simulink model "HeltonNonlinearProjectOne"  (R2018a)
settings: Solver=VariableStepAuto  StartTime=0.0  StopTime=100  MinStep=.001  RelTol=1e-5
settings Model: Creator=J  LastModifiedBy=J

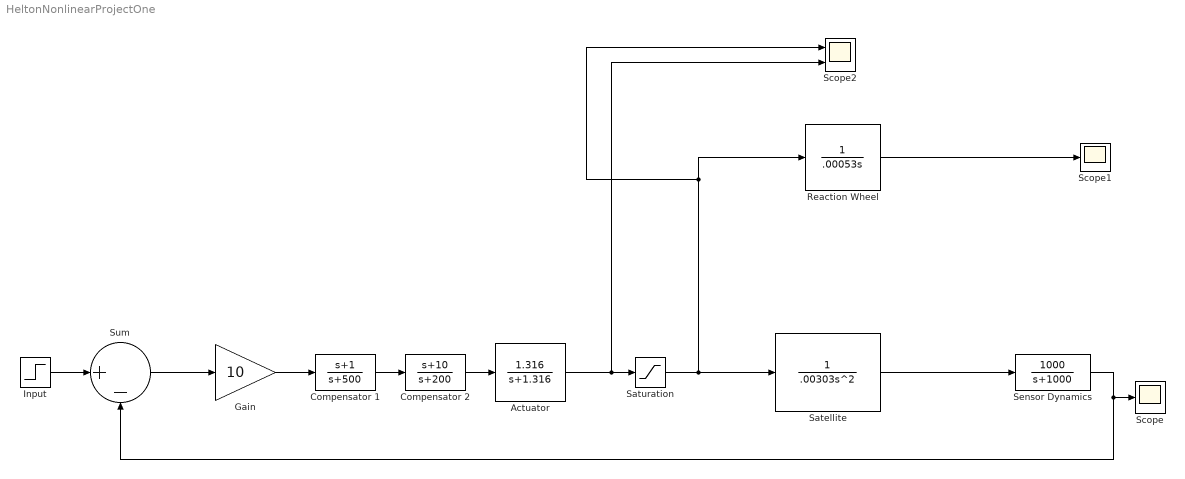
== system HeltonNonlinearProjectOne ==
  Actuator : TransferFcn  Numerator=[1.316]  Denominator=[1 1.316]
  Compensator 1 : TransferFcn  Numerator=[1 1]  Denominator=[1 500]
  Compensator 2 : TransferFcn  Numerator=[1 10]  Denominator=[1 200]
  Gain : Gain  Gain=10
  Input : Step  SampleTime=0
  Reaction Wheel : TransferFcn  Denominator=[.00053 0]
  Satellite : TransferFcn  Denominator=[.00303 0 0]
  Saturation : Saturate  UpperLimit=0.007  LowerLimit=-0.007
  Scope : Scope
  Scope1 : Scope
  Scope2 : Scope  NumInputPorts=2
  Sensor Dynamics : TransferFcn  Numerator=[1000]  Denominator=[1 1000]
  Sum : Sum  Inputs=|+-
  wires:
  Sum/1 -> Gain/1
  Input/1 -> Sum/1
  Reaction Wheel/1 -> Scope1/1
  Satellite/1 -> Sensor Dynamics/1
  Sensor Dynamics/1 -> Scope/1, Sum/2
  Gain/1 -> Compensator 1/1
  Compensator 2/1 -> Actuator/1
  Compensator 1/1 -> Compensator 2/1
  Saturation/1 -> Reaction Wheel/1, Scope2/1, Satellite/1
  Actuator/1 -> Saturation/1, Scope2/2
